simulink model "chap9_4sim"  (Simulink 7.7)
settings: Solver=ode45  StartTime=0.0  StopTime=40  FixedStep=0.001  RelTol=1e-3
settings Model: Creator=ljk  LastModifiedBy=ljk  ExtModeTrigMode=oneshot  ExtModeArmWhenConnect=off
settings DataIOCC: LimitDataPoints=off  SignalLoggingName=sigsOut
settings OptimizationCC: BooleanDataType=off
settings DebuggingCC: SaveWithParameterizedLinksMsg=none  SignalResolutionControl=TryResolveAllWithWarning  SolverPrmCheckMsg=none  MultiTaskDSMMsg=warning  MultiTaskCondExecSysMsg=none  StrictBusMsg=None
settings HardwareCC: TargetUnknown=on
settings RTWCC: IncludeERTFirstTime=on

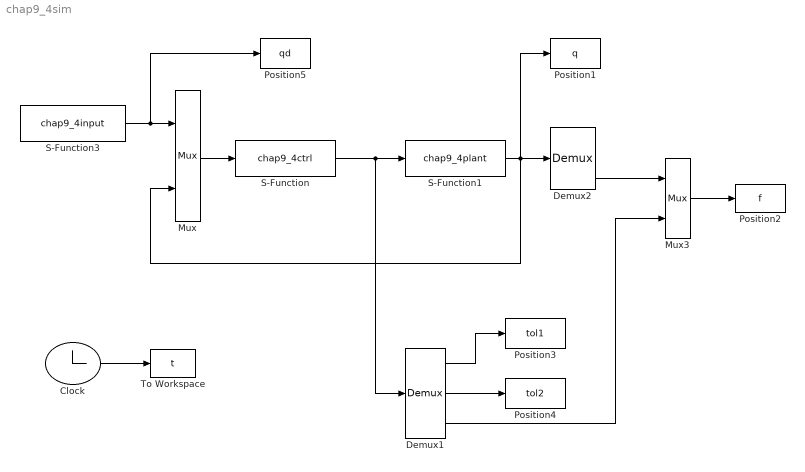
== system chap9_4sim ==
  Clock : Clock
      settings: Decimation=10
  Demux1 : Demux  Outputs=3
  Demux2 : Demux  Outputs=5
  Mux : Mux  Inputs=2
  Mux3 : Mux  Inputs=2
  Position1 : ToWorkspace  VariableName=q  SampleTime=-1  SaveFormat=Array
  Position2 : ToWorkspace  VariableName=f  SampleTime=-1  SaveFormat=Array
  Position3 : ToWorkspace  VariableName=tol1  SampleTime=-1  SaveFormat=Array
  Position4 : ToWorkspace  VariableName=tol2  SampleTime=-1  SaveFormat=Array
  Position5 : ToWorkspace  VariableName=qd  SampleTime=-1  SaveFormat=Array
  S-Function : S-Function  FunctionName=chap9_4ctrl  EnableBusSupport=off
  S-Function1 : S-Function  FunctionName=chap9_4plant  EnableBusSupport=off
  S-Function3 : S-Function  FunctionName=chap9_4input  EnableBusSupport=off
  To Workspace : ToWorkspace  VariableName=t  SampleTime=-1  SaveFormat=Array
  wires:
  Mux/1 -> S-Function/1
  S-Function1/1 -> Demux2/1, Mux/2, Position1/1
  Demux1/1 -> Position3/1
  Demux1/2 -> Position4/1
  S-Function/1 -> S-Function1/1, Demux1/1
  Mux3/1 -> Position2/1
  Demux1/3 -> Mux3/2
  Demux2/5 -> Mux3/1
  Clock/1 -> To Workspace/1
  S-Function3/1 -> Mux/1, Position5/1
